simulink model "essai"  (R2016b)
settings: Solver=FixedStepAuto  StartTime=0.0  StopTime=40.0  FixedStep=0.001  RelTol=1e-3
settings Model: Creator=vanou  LastModifiedBy=vanou

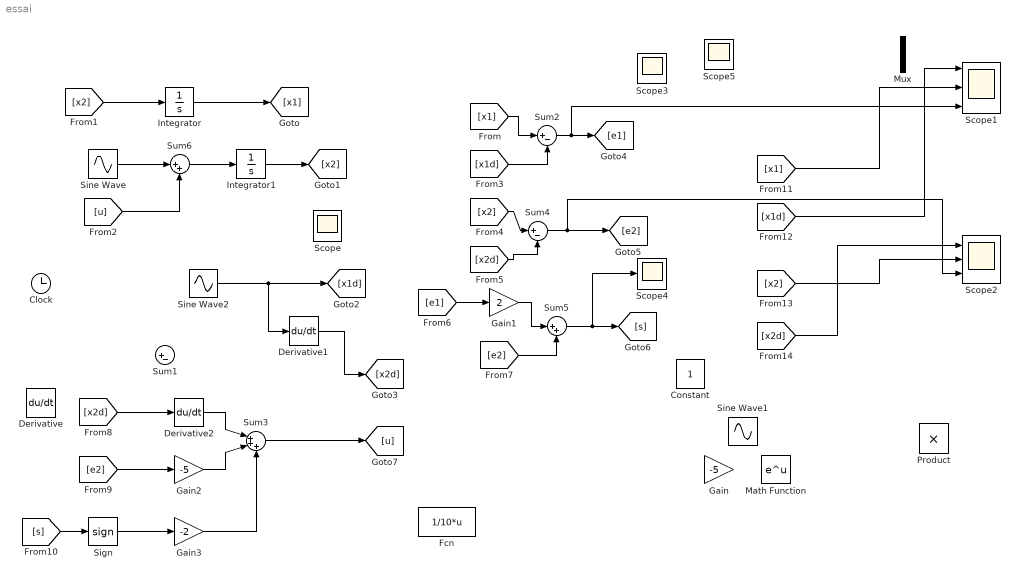
== system essai ==
  Clock : Clock
  Constant : Constant
  Derivative : Derivative
  Derivative1 : Derivative
  Derivative2 : Derivative
  Fcn : Fcn  Expr=1/10*u
  Gain : Gain  Gain=-5
  Gain1 : Gain  Gain=2
  Gain2 : Gain  Gain=-5
  Gain3 : Gain  Gain=-2
  Integrator : Integrator  InitialCondition=1
  Integrator1 : Integrator
  Math Function : Math  SaturateOnIntegerOverflow=on
  Mux : Mux  Inputs=2
  Product : Product
  Scope{,3..5} (4 alike) : Scope
  Scope1 : Scope  NumInputPorts=3
  Scope2 : Scope  NumInputPorts=3
  Sign : Signum
  Sine Wave : Sin  SampleTime=0
  Sine Wave1 : Sin  SampleTime=0
  Sine Wave2 : Sin  SampleTime=0
  Sum1 : Sum  Inputs=|+-
  Sum2 : Sum  Inputs=|+-
  Sum3 : Sum  Inputs=|+++
  Sum4 : Sum  Inputs=|+-
  Sum5 : Sum  Inputs=|++
  Sum6 : Sum  Inputs=|++
  wires:
  [x2] -> Integrator/1
  Integrator/1 -> [x1]
  Sum6/1 -> Integrator1/1
  Integrator1/1 -> [x2]
  [u] -> Sum6/2
  [x1] -> Sum2/1
  [x1d] -> Sum2/2
  Sum2/1 -> Scope1/3, [e1]
  [x2] -> Sum4/1
  [x2d] -> Sum4/2
  Sum4/1 -> Scope2/3, [e2]
  [e2] -> Sum5/2
  Sum5/1 -> Scope4/1, [s]
  [e1] -> Gain1/1
  Gain1/1 -> Sum5/1
  [e2] -> Gain2/1
  [x2d] -> Derivative2/1
  Sum3/1 -> [u]
  Derivative2/1 -> Sum3/1
  Gain3/1 -> Sum3/3
  Gain2/1 -> Sum3/2
  Sign/1 -> Gain3/1
  [s] -> Sign/1
  Sine Wave/1 -> Sum6/1
  [x2] -> Scope2/2
  [x2d] -> Scope2/1
  [x1d] -> Scope1/1
  [x1] -> Scope1/2
  Derivative1/1 -> [x2d]
  Sine Wave2/1 -> Derivative1/1, [x1d]
